simulink model "TransmissionController"  (R2026a)
settings: Solver=FixedStepAuto  StopTime=65  FixedStep=0.5
undefined symbols (not defined in the file): RangeSelected
libraries: simulink x6, sl_discontinuities x1
settings Model: DataDictionary=ETRS_data.sldd  Creator=macec  LastModifiedBy=anna

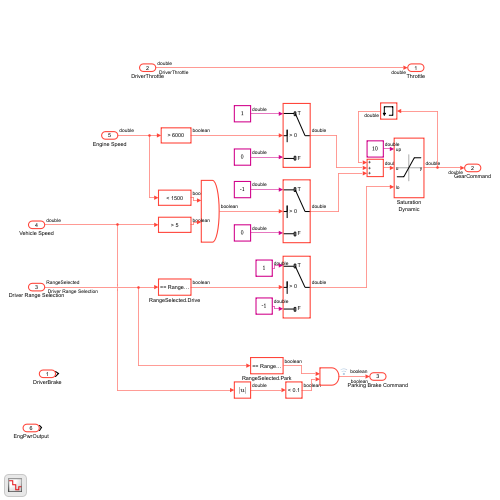
[thumbnail: Simulink's stored preview of the top-level diagram]
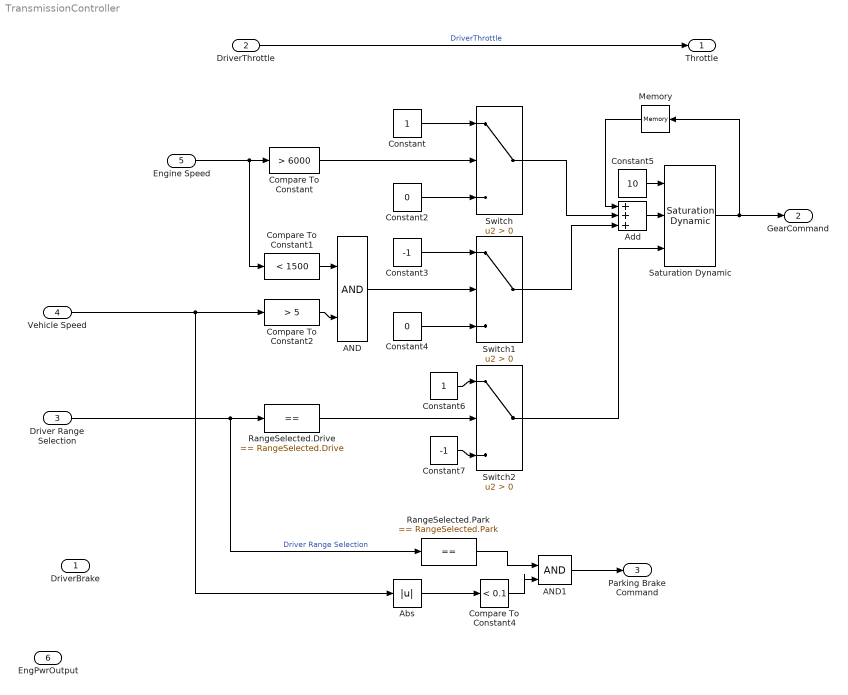
== system TransmissionController ==
  DriverBrake : Inport  OutDataTypeStr=double  PortDimensions=1
  DriverThrottle : Inport  Port=2  OutDataTypeStr=double  PortDimensions=1
  Driver Range Selection : Inport  Port=3  OutDataTypeStr=Enum: RangeSelected  PortDimensions=1
  Vehicle Speed : Inport  Port=4  OutDataTypeStr=double  PortDimensions=1
  Engine Speed : Inport  Port=5  OutDataTypeStr=double  PortDimensions=1
  EngPwrOutput : Inport  Port=6
  AND : Logic  IconShape=distinctive  AllPortsSameDT=off  OutDataTypeStr=boolean
  AND1 : Logic  IconShape=distinctive  AllPortsSameDT=off  OutDataTypeStr=boolean
  Abs : Abs  SaturateOnIntegerOverflow=off
  Add : Sum  Inputs=+++
  Compare To Constant : simulink/Logic and Bit Operations/Compare To Constant  relop=>  const=6000  OutDataTypeStr=boolean
  Compare To Constant1 : simulink/Logic and Bit Operations/Compare To Constant  relop=<  const=1500  OutDataTypeStr=boolean
  Compare To Constant2 : simulink/Logic and Bit Operations/Compare To Constant  relop=>  const=5  OutDataTypeStr=boolean
  Compare To Constant4 : simulink/Logic and Bit Operations/Compare To Constant  relop=<  const=0.1  OutDataTypeStr=boolean
  Constant : Constant
  Constant2 : Constant  Value=0
  Constant3 : Constant  Value=-1
  Constant4 : Constant  Value=0
  Constant5 : Constant  Value=10
  Constant6 : Constant
  Constant7 : Constant  Value=-1
  Memory : Memory  InheritSampleTime=on
  RangeSelected.Drive : simulink/Logic and Bit Operations/Compare To Constant  relop===  const=RangeSelected.Drive  OutDataTypeStr=boolean
  RangeSelected.Park : simulink/Logic and Bit Operations/Compare To Constant  relop===  const=RangeSelected.Park  OutDataTypeStr=boolean
  Saturation Dynamic : sl_discontinuities/Saturation Dynamic  OutMin=[]  OutMax=[]  OutDataTypeStr=Inherit: Same as second input  OutDataType=fixdt(1, 16)  OutScaling=2^-10  DoSatur=off
      settings: LibrarySourceBlock=|
      | simulink/Discontinuities/Saturation
      | Dynamic
  Switch : Switch  Criteria=u2 > Threshold  SaturateOnIntegerOverflow=off  InputSameDT=off
  Switch1 : Switch  Criteria=u2 > Threshold  SaturateOnIntegerOverflow=off  InputSameDT=off
  Switch2 : Switch  Criteria=u2 > Threshold  SaturateOnIntegerOverflow=off  InputSameDT=off
  Throttle : Outport  OutDataTypeStr=double  PortDimensions=1
  GearCommand : Outport  Port=2  OutDataTypeStr=double  PortDimensions=1
  Parking Brake Command : Outport  Port=3  OutDataTypeStr=boolean  PortDimensions=1
  wires:
  Engine Speed/1 -> Compare To Constant/1, Compare To Constant1/1
  Compare To Constant/1 -> Switch/2
  Constant/1 -> Switch/1
  Constant2/1 -> Switch/3
  Constant3/1 -> Switch1/1
  Constant4/1 -> Switch1/3
  Compare To Constant2/1 -> AND/2
  AND/1 -> Switch1/2
  Compare To Constant1/1 -> AND/1
  Saturation Dynamic/1 -> GearCommand/1, Memory/1
  Switch1/1 -> Add/3
  Switch/1 -> Add/2
  Memory/1 -> Add/1
  Constant5/1 -> Saturation Dynamic/1
  Add/1 -> Saturation Dynamic/2
  RangeSelected.Drive/1 -> Switch2/2
  Constant6/1 -> Switch2/1
  Constant7/1 -> Switch2/3
  Switch2/1 -> Saturation Dynamic/3
  DriverThrottle/1 -> Throttle/1  "DriverThrottle"
  Driver Range Selection/1 -> RangeSelected.Park/1, RangeSelected.Drive/1  "Driver Range Selection"
  Vehicle Speed/1 -> Abs/1, Compare To Constant2/1
  Abs/1 -> Compare To Constant4/1
  Compare To Constant4/1 -> AND1/2
  RangeSelected.Park/1 -> AND1/1
  AND1/1 -> Parking Brake Command/1
